simulink model "MODEL_GR2_WITH_BRAKKING"  (R2023b)
settings: Solver=VariableStepAuto  StartTime=0.0  StopTime=T_tot  RelTol=1e-3
values from neighbouring files (symbols this model uses):
  B = 0.0129    [PARAMETERS_MODEL_GR2.m]    (also in Parameters.m; Parameters_Chloe.m)
  C_dc = 15e-3    (= 0.015)    [PARAMETERS_MODEL_GR2.m]    (also in Parameters.m; Parameters_Chloe.m)
  f_grid = 50    [PARAMETERS_MODEL_GR2.m]    (also in Parameters.m; Parameters_Chloe.m)
  f_r = 50    [PARAMETERS_MODEL_GR2.m]    (also in Parameters.m; Parameters_Chloe.m)
  J = 0.2799    [PARAMETERS_MODEL_GR2.m]    (also in Parameters.m; Parameters_Chloe.m)
  Ki = Ki*Ts_w    (= 0.00645)    [PARAMETERS_MODEL_GR2.m]    (also in Parameters.m = 0.37903125; Parameters_Chloe.m = 1.04185)
  Kp = Kp + Ki*Ts_w/2    (= 210.627975)    [PARAMETERS_MODEL_GR2.m]    (also in Parameters.m = 2.463703125; Parameters_Chloe.m = 6.772025)
  L_grid = 1.5e-6    (= 1.5e-06)    [PARAMETERS_MODEL_GR2.m]    (also in Parameters.m = 2e-05; Parameters_Chloe.m = 2e-05)
  L_lr = 1.8e-3    (= 0.0018)    [PARAMETERS_MODEL_GR2.m]    (also in Parameters.m; Parameters_Chloe.m)
  L_ls = 1.8e-3    (= 0.0018)    [PARAMETERS_MODEL_GR2.m]    (also in Parameters.m; Parameters_Chloe.m)
  L_rectif = 10e-3    (= 0.01)    [PARAMETERS_MODEL_GR2.m]    (also in Parameters.m; Parameters_Chloe.m)
  N_steady = N_r    (= 1460)    [PARAMETERS_MODEL_GR2.m]    (also in Parameters.m = 1450; Parameters_Chloe.m = 1450)
  P = 4    [PARAMETERS_MODEL_GR2.m]    (also in Parameters.m; Parameters_Chloe.m)
  p = P/2    (= 2)    [PARAMETERS_MODEL_GR2.m]
  P_r = 19e3    (= 19000)    [PARAMETERS_MODEL_GR2.m]    (also in Parameters.m; Parameters_Chloe.m)
  Phi_n = V_s/w_s    [PARAMETERS_MODEL_GR2.m]    (also in Parameters.m = V_r*sqrt(2)/sqrt(3)/(2*pi*f_r); Parameters_Chloe.m = V_r*sqrt(2)/sqrt(3)/(2*pi*f_r))
  R_grid = 0.005    [PARAMETERS_MODEL_GR2.m]    (also in Parameters.m = 0.2; Parameters_Chloe.m = 0.2)
  R_r = 0.1091    [PARAMETERS_MODEL_GR2.m]    (also in Parameters.m; Parameters_Chloe.m)
  R_s = 0.0629    [PARAMETERS_MODEL_GR2.m]    (also in Parameters.m; Parameters_Chloe.m)
  Slope_down = -N_steady/(t_rampdown_end - t_rampdown_start)    (= -912.5)    [PARAMETERS_MODEL_GR2.m]
  Slope_up = N_steady/(t_rampup_end - t_rampup_start)    (= 912.5)    [PARAMETERS_MODEL_GR2.m]
  t_delay_down = 0.01*T_tot    (= 0.08)    [PARAMETERS_MODEL_GR2.m]
  t_delay_up = 0.03*T_tot    (= 0.24)    [PARAMETERS_MODEL_GR2.m]
  T_load = 0.8*T_r    (= 99.4173343149)    [PARAMETERS_MODEL_GR2.m]
  t_rampdown_end = 0.95*T_tot    (= 7.6)    [PARAMETERS_MODEL_GR2.m]
  t_rampdown_start = 0.75*T_tot    (= 6)    [PARAMETERS_MODEL_GR2.m]
  t_rampup_start = 0.05*T_tot    (= 0.4)    [PARAMETERS_MODEL_GR2.m]
  T_sat = 0.9*T_max    [PARAMETERS_MODEL_GR2.m]    (also in Parameters.m = 124.271667894; Parameters_Chloe.m = 621.358339468)
  Ts = 5e-6    (= 5e-06)    [PARAMETERS_MODEL_GR2.m]    (also in Parameters.m = 1e-05; Parameters_Chloe.m = 1e-05)
  Ts_w = 1/fs_w    (= 0.000664451827243)    [PARAMETERS_MODEL_GR2.m]    (also in Parameters.m = 0.0410256410256; Parameters_Chloe.m = 0.0149253731343)
  U_ac = 380    [PARAMETERS_MODEL_GR2.m]    (also in Parameters.m; Parameters_Chloe.m)
  V_f_in = [-f_r-1 -f_r -f_min 0 f_min f_r f_r+1]*2*pi    [PARAMETERS_MODEL_GR2.m]    (also in Parameters.m; Parameters_Chloe.m)
  V_f_out = [V_s V_s V_min V_min V_min V_s V_s]/V_s    [PARAMETERS_MODEL_GR2.m]    (also in Parameters.m = [V_r V_r V_min V_min V_min V_r V_r]/V_r; Parameters_Chloe.m = [V_r V_r V_min V_min V_min V_r V_r]/V_r)
  V_r = 400    [PARAMETERS_MODEL_GR2.m]    (also in Parameters.m; Parameters_Chloe.m)
libraries: spsDiodeLib x13, spsIGBTLib x7, spsSeriesRLCBranchLib x6, spsACVoltageSourceLib x3, spsThreePhaseVIMeasurementLib x3, spsMeanLib x2, spsRMSLib x2, simulink x2, spsAsynchronousMachineSIUnitsLib x1, spsCurrentMeasurementLib x1, spsGroundLib x1, spsThreePhaseTransformerTwoWindingsLib x1
settings Model: Creator=dimit  LastModifiedBy=User

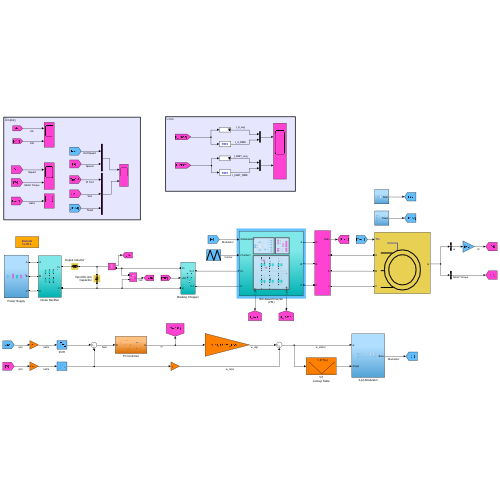
[thumbnail: Simulink's stored preview of the top-level diagram]
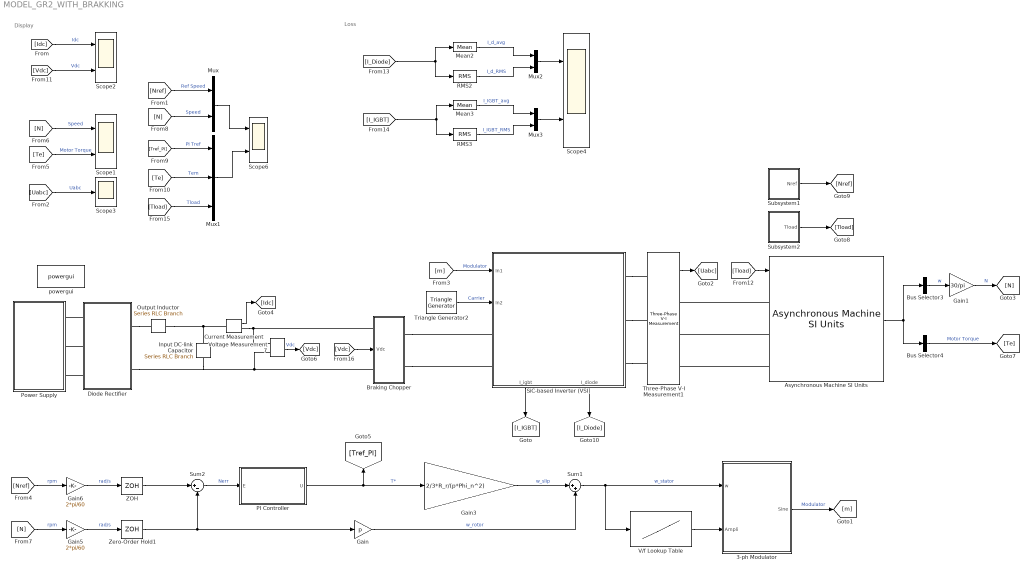
== system MODEL_GR2_WITH_BRAKKING ==
  note: Display
  note: Loss
  3-ph Modulator : Subsystem
  Asynchronous Machine SI Units : spsAsynchronousMachineSIUnitsLib/Asynchronous Machine SI Units  RotorType=Squirrel-cage  PresetModel=No  MechanicalLoad=Torque Tm  ShowDetailedParameters=on  ReferenceFrame=Rotor  Units=SI  MeasurementBus=off  NominalParameters=[P_r V_r f_r]  VoltageRatio=1  Stator=[R_s L_ls]  Rotor=[R_r L_lr]  Cage1=[0.4155 0.002066]  Cage2=[0.4168 0.0003495]  Lm=L_m  Mechanical=[J B P/2]  PolePairs=2  InitialConditions=[1 0 0 0 0 0 0 0]  SimulateSaturation=off  Saturation=[14.03593122, 27.81365428, 53.79336849, 72.68890987, 97.98006896, 148.6815601, 215.7428561, 302.9841135, 428.7778367 ; 230, 322, 414, 460, 506, 552, 598, 644, 690]  LoadFlowParameters=1492000  TsPowergui=0  TsBlock=-1  IterativeModel=Trapezoidal non iterative  IterativeDiscreteModel=Trapezoidal non iterative  Pmec=1.492e+006
  Braking Chopper : Subsystem
      settings: PortSchema="{\"entries\":[{\"content\":{\"sides\":[{\"content\":{\"connectorIds\":[\"LConn1\",\"In1\",\"LConn2\"]},\"type\":\"ConnectorPlacement.EquallySpacedRectSide\",\"uuid\":\"08066bb6-7173-482b-b457-6e49107a8511\"},{\"content\":{\"connectorIds\":[\"RConn1\",\"RConn2\"],\"side\":\"RIGHT\"},\"type\":\"ConnectorPlacement.EquallySpacedRectSide\",\"uuid\":\"28fab536-82b6-47c9-b368-73f431d395c4\"},{\"content\":{\"side\":\"TOP\"},\"type\":\"ConnectorPlacement.EquallySpacedRectSide\",\"uuid\":\"9838844e-a39c-4f91-95c1-e91ef715e2ab\"}]},\"type\":\"ConnectorPlacement.EquallySpacedConnector\",\"uuid\":\"fe40f05d-eb20-40bd-af99-b051ef6fbc42\"}],\"packageUris\":[\"http://schema.mathworks.com/mf0/Connector/R2020b\"],\"version\":\"1.0\"}"
  Bus Selector3 : BusSelector  OutputSignals=Mechanical.Rotor speed (wm)  OutputAsBus=on
  Bus Selector4 : BusSelector  OutputSignals=Mechanical.Electromagnetic torque Te (N*m)  OutputAsBus=on
  Current Measurement : spsCurrentMeasurementLib/Current Measurement  PhasorSimulation=off  OutputType=Complex  PSBequivalent=0
  Diode Rectifier : Subsystem
  Gain : Gain  Gain=p
  Gain1 : Gain  Gain=30/pi
  Gain3 : Gain  Gain=2/3*R_r/(p*Phi_n^2)
  Gain5 : Gain  Gain=2*pi/60
  Gain6 : Gain  Gain=2*pi/60
  Input DC-link Capacitor : spsSeriesRLCBranchLib/Series RLC Branch  LConnTagsString=__new0  RConnTagsString=__new0  BranchType=C  Resistance=1  Inductance=1e-3  SetiL0=off  InitialCurrent=0  Capacitance=C_dc  Setx0=off  InitialVoltage=0  Measurements=None
  Mean2 : spsMeanLib/Mean  Freq=10  Vinit=0  Ts=Ts
  Mean3 : spsMeanLib/Mean  Freq=10  Vinit=0  Ts=Ts
  Mux : Mux  Inputs=2
  Mux1 : Mux  Inputs=3
  Mux2 : Mux  Inputs=2
  Mux3 : Mux  Inputs=2
  Output Inductor : spsSeriesRLCBranchLib/Series RLC Branch  LConnTagsString=__new0  RConnTagsString=__new0  BranchType=L  Resistance=1  Inductance=L_rectif  SetiL0=off  InitialCurrent=0  Capacitance=15e-6  Setx0=off  InitialVoltage=0  Measurements=None
  PI Controller : Subsystem
  Power Supply : Subsystem
  RMS2 : spsRMSLib/RMS  TrueRMS=on  Freq=10  RMSInit=0  Ts=Ts
  RMS3 : spsRMSLib/RMS  TrueRMS=on  Freq=10  RMSInit=0  Ts=Ts
  Scope{1..2,4,6} (4 alike) : Scope  NumInputPorts=2
  Scope3 : Scope
  SiC-based Inverter (VSI) : Subsystem
      settings: PortSchema="{\"entries\":[{\"content\":{\"sides\":[{\"content\":{\"connectorIds\":[\"In1\",\"In2\",\"LConn1\",\"LConn2\"]},\"type\":\"ConnectorPlacement.EquallySpacedRectSide\",\"uuid\":\"45fc5859-179e-40d9-92a1-bdc86f2558ba\"},{\"content\":{\"connectorIds\":[\"RConn1\",\"RConn2\",\"RConn3\"],\"side\":\"RIGHT\"},\"type\":\"ConnectorPlacement.EquallySpacedRectSide\",\"uuid\":\"a0d57c1e-c527-4dbd-a036-7c0d4c1ba50f\"},{\"content\":{\"side\":\"TOP\"},\"type\":\"ConnectorPlacement.EquallySpacedRectSide\",\"uuid\":\"ae8306ed-bce6-46bd-8f47-d4ecdbdade45\"},{\"content\":{\"connectorIds\":[\"Out1\",\"Out2\"],\"side\":\"BOTTOM\"},\"type\":\"ConnectorPlacement.EquallySpacedRectSide\",\"uuid\":\"956e186d-7720-45d4-9cd3-94ca775912d4\"}]},\"type\":\"ConnectorPlacement.EquallySpacedConnector\",\"uuid\":\"758af6d4-83da-4acf-a819-436e3391a35e\"}],\"packageUris\":[\"http://schema.mathworks.com/mf0/Connector/R2020b\"],\"version\":\"1.0\"}"
  Subsystem1 : Subsystem
  Subsystem2 : Subsystem
  Sum1 : Sum  Inputs=|++
  Sum2 : Sum  Inputs=|+-
  Three-Phase V-I Measurement1 : spsThreePhaseVIMeasurementLib/Three-Phase V-I Measurement  VoltageMeasurement=phase-to-phase  SetLabelV=off  LabelV=Vabc  Vpu=off  VpuLL=off  CurrentMeasurement=no  SetLabelI=off  LabelI=Iabc  Ipu=off  Pbase=100e6  Vbase=500e3  OutputType=Complex  PhasorSimulation=off  PSBequivalent=0
  Triangle Generator2 : spsTriangleGeneratorLib/Triangle Generator  Freq=f_switch  Phase=0  Ts=0
  V/f Lookup Table : Lookup_n-D  NumberOfTableDimensions=1  BreakpointsForDimension1=V_f_in  Table=V_f_out  InternalRulePriority=Speed  RndMeth=Simplest
  Voltage Measurement7 : spsVoltageMeasurementLib/Voltage Measurement  PhasorSimulation=off  OutputType=Complex  PSBequivalent=0
  ZOH : ZeroOrderHold  SampleTime=Ts_w
  Zero-Order Hold1 : ZeroOrderHold  SampleTime=Ts_w
  powergui : spspowerguiLib/powergui  Priority=1  SimulationMode=Discrete  SampleTime=Ts  frequency=60  Iterations=50  frequencyindice=0  Pbase=100e6  ErrMax=1e-4  UnitsV=kV  UnitsW=MW  buscounter=0  FunctionMessages=off  echomessages=off  EnableUseOfTLC=off  CurrentSourceSwitches=off  DisableSnubberDevices=off  DisableRonSwitches=off  DisableVfSwitches=off  DisplayEquations=off  AutomaticDiscreteSolvers=off  SolverType=Tustin/Backward Euler (TBE)  Interpol=off  ExternalGateDelay=off  methode=off  Ts=100  x0status=blocks  SPID=on  SwTol=0  HookPort=off  NonlinearTolerance=1e-4  nMaxIteration=100  ContinueOnMaxIteration=off  RestoreLinks=warning  ResistiveCurrentMeasurement=off  Frange=[0:2:500]  Ylog=off  Xlog=on  ShowGrid=off  save=off  variable=ZData  structure=0  ZoomFFT=off  StartTime=0.0  cycles=1  DisplayStyle=1  fundamental=60  FreqAxis=off  MaxFrequency=1000  frequencyindicesteady=1  RmsSteady=1  display=off
  wires:
  [Te] -> Mux1/2  "Tem"
  Gain1/1 -> [N]  "N"
  [m] -> SiC-based Inverter (VSI)/1(In1)  "Modulator"
  [Uabc] -> Scope3/1  "Uabc"
  [Tref_PI] -> Mux1/1  "PI Tref"
  [Te] -> Scope1/2  "Motor Torque"
  Three-Phase V-I Measurement1/1 -> [Uabc]
  [Nref] -> Mux/1  "Ref Speed"
  [N] -> Mux/2  "Speed"
  Mux1/1 -> Scope6/2
  Triangle Generator2/1 -> SiC-based Inverter (VSI)/2(In2)  "Carrier"
  Mux/1 -> Scope6/1
  [N] -> Scope1/1  "Speed"
  Asynchronous Machine SI Units/1 -> Bus Selector3/1, Bus Selector4/1
  Bus Selector3/1 -> Gain1/1  "w"
  Bus Selector4/1 -> [Te]  "Motor Torque"
  Current Measurement/1 -> [Idc]
  Voltage Measurement7/1 -> [Vdc]  "Vdc"
  [Idc] -> Scope2/1  "Idc"
  [Vdc] -> Scope2/2  "Vdc"
  SiC-based Inverter (VSI)/1(I_igbt) -> [I_IGBT]
  PI Controller/1(U) -> [Tref_PI], Gain3/1  "T*"
  Sum1/1 -> V/f Lookup Table/1, 3-ph Modulator/1(w)  "w_stator"
  Zero-Order Hold1/1 -> Sum2/2, Gain/1
  ZOH/1 -> Sum2/1
  V/f Lookup Table/1 -> 3-ph Modulator/2(Ampli)
  [N] -> Gain5/1  "rpm"
  Gain6/1 -> ZOH/1  "rad/s"
  3-ph Modulator/1(Sine) -> [m]  "Modulator"
  Gain3/1 -> Sum1/1  "w_slip"
  Gain/1 -> Sum1/2  "w_rotor"
  Gain5/1 -> Zero-Order Hold1/1  "rad/s"
  [Nref] -> Gain6/1  "rpm"
  Sum2/1 -> PI Controller/1(E)  "Nerr"
  [Tload] -> Asynchronous Machine SI Units/1
  [I_IGBT] -> RMS3/1, Mean3/1
  Mean2/1 -> Mux2/1  "I_d_avg"
  Mean3/1 -> Mux3/1  "I_IGBT_avg"
  [I_Diode] -> Mean2/1, RMS2/1
  RMS2/1 -> Mux2/2  "I_d_RMS"
  SiC-based Inverter (VSI)/2(I_diode) -> [I_Diode]
  Subsystem2/1(Tload) -> [Tload]
  Subsystem1/1(Nref) -> [Nref]
  [Tload] -> Mux1/3  "Tload"
  RMS3/1 -> Mux3/2  "I_IGBT_RMS"
  Mux2/1 -> Scope4/1
  Mux3/1 -> Scope4/2
  [Vdc] -> Braking Chopper/1(Vdc)
  connections:
  SiC-based Inverter (VSI)/RConn1 -- Three-Phase V-I Measurement1/LConn1
  Asynchronous Machine SI Units/LConn3 -- Three-Phase V-I Measurement1/RConn3
  SiC-based Inverter (VSI)/RConn3 -- Three-Phase V-I Measurement1/LConn3
  Asynchronous Machine SI Units/LConn1 -- Three-Phase V-I Measurement1/RConn1
  SiC-based Inverter (VSI)/RConn2 -- Three-Phase V-I Measurement1/LConn2
  Asynchronous Machine SI Units/LConn2 -- Three-Phase V-I Measurement1/RConn2
  Input DC-link Capacitor/RConn1 -- Diode Rectifier/RConn2 -- Braking Chopper/LConn2 -- Voltage Measurement7/LConn2
  Current Measurement/RConn1 -- Voltage Measurement7/LConn1 -- Braking Chopper/LConn1
  Output Inductor/LConn1 -- Input DC-link Capacitor/LConn1 -- Current Measurement/LConn1
  Diode Rectifier/LConn1 -- Power Supply/LConn1
  Diode Rectifier/LConn2 -- Power Supply/LConn2
  Diode Rectifier/RConn1 -- Output Inductor/RConn1
  Diode Rectifier/LConn3 -- Power Supply/LConn3
  Braking Chopper/RConn1 -- SiC-based Inverter (VSI)/LConn1
  Braking Chopper/RConn2 -- SiC-based Inverter (VSI)/LConn2

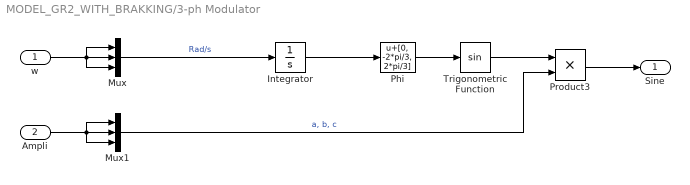
== system MODEL_GR2_WITH_BRAKKING/3-ph Modulator ==
  w : Inport
  Ampli : Inport  Port=2
  Integrator : Integrator
  Mux : Mux  Inputs=3
  Mux1 : Mux  Inputs=3
  Phi : Bias  Bias=[0, -2*pi/3, 2*pi/3]  SaturateOnIntegerOverflow=off
  Product3 : Product
  Trigonometric Function : Trigonometry
  Sine : Outport
  wires:
  Integrator/1 -> Phi/1
  Trigonometric Function/1 -> Product3/1
  Mux/1 -> Integrator/1  "Rad/s"
  Mux1/1 -> Product3/2  "a, b, c"
  Ampli/1 -> Mux1/1, Mux1/3, Mux1/2
  w/1 -> Mux/3, Mux/2, Mux/1
  Phi/1 -> Trigonometric Function/1
  Product3/1 -> Sine/1

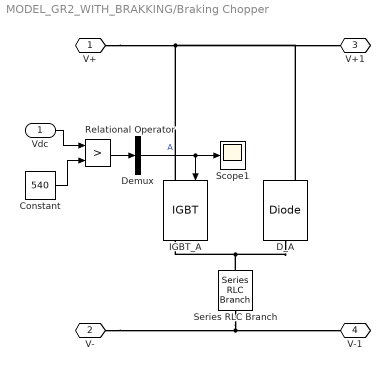
== system MODEL_GR2_WITH_BRAKKING/Braking Chopper ==
  Vdc : Inport
  Constant : Constant  Value=540
  D_A : spsDiodeLib/Diode  Ron=R_d_inv  Lon=L_on_inv  Vf=V_f_inv  IC=0  UseSnubber=0  Rs=R_snub_inv  Cs=C_snub_inv  Measurements=on
  Demux : Demux  Outputs=1
  IGBT_A : spsIGBTLib/IGBT  Ron=R_on_inv  Lon=L_on_inv  Vf=V_f_inv  Tf=1e-6  Tt=2e-6  IC=0  Rs=R_snub_inv  Cs=C_snub_inv  Measurements=on
  Relational Operator : RelationalOperator  Operator=>  OutDataTypeStr=boolean  RndMeth=Simplest  InputSameDT=off
  Scope1 : Scope
  Series RLC Branch : spsSeriesRLCBranchLib/Series RLC Branch  LConnTagsString=__new0  RConnTagsString=__new0  BranchType=R  Resistance=20  Inductance=1e-3  SetiL0=off  InitialCurrent=0  Capacitance=1e-6  Setx0=off  InitialVoltage=0  Measurements=None
  V+ : PMIOPort  Side=Left
  V- : PMIOPort  Port=2  Side=Left
  V+1 : PMIOPort  Port=3  Side=Right
  V-1 : PMIOPort  Port=4  Side=Right
  wires:
  Vdc/1 -> Relational Operator/1
  Constant/1 -> Relational Operator/2
  Relational Operator/1 -> Demux/1
  Demux/1 -> Scope1/1, IGBT_A/1  "A"
  connections:
  V+/RConn1 -- IGBT_A/LConn1 -- D_A/RConn1 -- V+1/RConn1
  V-/RConn1 -- Series RLC Branch/RConn1 -- V-1/RConn1
  Series RLC Branch/LConn1 -- D_A/LConn1 -- IGBT_A/RConn1

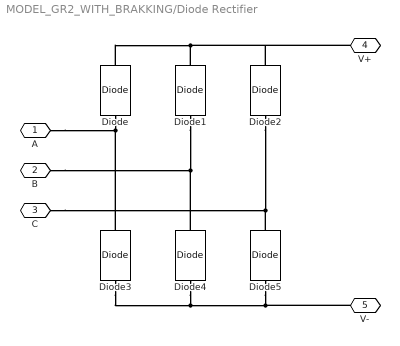
== system MODEL_GR2_WITH_BRAKKING/Diode Rectifier ==
  Diode{,1..5} (6 alike) : spsDiodeLib/Diode  Ron=R_on_rect  Lon=0  Vf=V_f_rect  IC=0  UseSnubber=0  Rs=R_snub_rect  Cs=C_snub_rect  Measurements=off
  A : PMIOPort  Side=Left
  B : PMIOPort  Port=2  Side=Left
  C : PMIOPort  Port=3  Side=Left
  V+ : PMIOPort  Port=4  Side=Right
  V- : PMIOPort  Port=5  Side=Right
  connections:
  B/RConn1 -- Diode4/RConn1 -- Diode1/LConn1
  Diode4/LConn1 -- Diode3/LConn1 -- Diode5/LConn1 -- V-/RConn1
  C/RConn1 -- Diode5/RConn1 -- Diode2/LConn1
  Diode/LConn1 -- Diode3/RConn1 -- A/RConn1
  Diode/RConn1 -- Diode1/RConn1 -- Diode2/RConn1 -- V+/RConn1

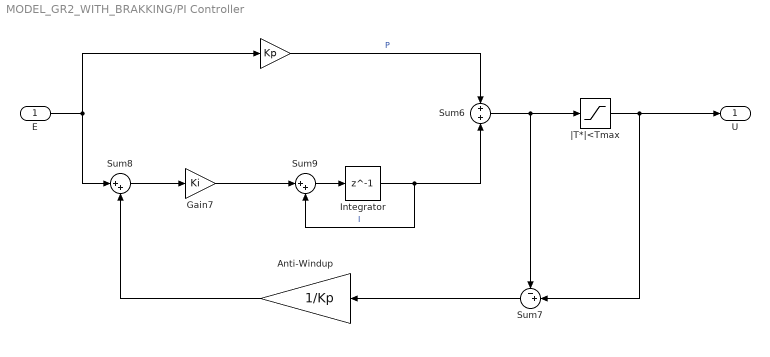
== system MODEL_GR2_WITH_BRAKKING/PI Controller ==
  E : Inport
  " " : Gain  Gain=Kp
  Anti-Windup : Gain  Gain=1/Kp
  Gain7 : Gain  Gain=Ki
  Integrator : Delay  DelayLength=1  SampleTime=Ts_w
  Sum6 : Sum
  Sum7 : Sum  Inputs=-+|
  Sum8 : Sum  Inputs=|++
  Sum9 : Sum  Inputs=|++
  |T*|<Tmax : Saturate  UpperLimit=T_sat  LowerLimit=-T_sat
  U : Outport
  wires:
  Sum8/1 -> Gain7/1
  Anti-Windup/1 -> Sum8/2
  E/1 -> Sum8/1, " "/1
  Sum6/1 -> |T*|<Tmax/1, Sum7/1
  " "/1 -> Sum6/1  "P"
  |T*|<Tmax/1 -> Sum7/2, U/1
  Integrator/1 -> Sum6/2, Sum9/2  "I"
  Sum7/1 -> Anti-Windup/1
  Gain7/1 -> Sum9/1
  Sum9/1 -> Integrator/1

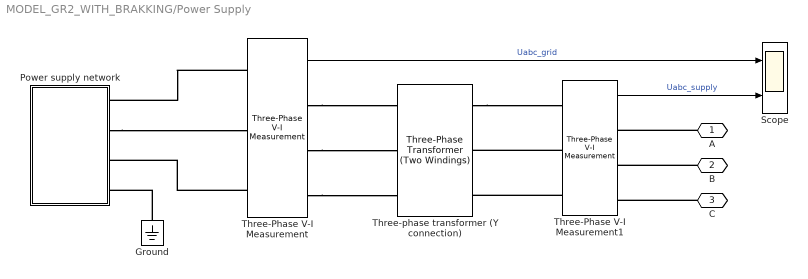
== system MODEL_GR2_WITH_BRAKKING/Power Supply ==
  Ground : spsGroundLib/Ground  LConnTagsString=a
  Power supply network : Subsystem
  Scope : Scope  NumInputPorts=2
  Three-Phase V-I Measurement : spsThreePhaseVIMeasurementLib/Three-Phase V-I Measurement  VoltageMeasurement=phase-to-phase  SetLabelV=off  LabelV=Vabc  Vpu=off  VpuLL=off  CurrentMeasurement=no  SetLabelI=off  LabelI=Iabc  Ipu=off  Pbase=100e6  Vbase=500e3  OutputType=Complex  PhasorSimulation=off  PSBequivalent=0
  Three-Phase V-I Measurement1 : spsThreePhaseVIMeasurementLib/Three-Phase V-I Measurement  VoltageMeasurement=phase-to-phase  SetLabelV=off  LabelV=Vabc  Vpu=off  VpuLL=off  CurrentMeasurement=no  SetLabelI=off  LabelI=Iabc  Ipu=off  Pbase=100e6  Vbase=500e3  OutputType=Complex  PhasorSimulation=off  PSBequivalent=0
  Three-phase transformer (Y connection) : spsThreePhaseTransformerTwoWindingsLib/Three-Phase Transformer (Two Windings)  Winding1Connection=Y  Winding2Connection=Yg  CoreType=Three single-phase transformers  SetSaturation=off  Hysteresis=off  DataFile='hysteresis'  SetInitialFlux=off  Measurements=None  UNITS=pu  NominalPower=[ 20e3 , 50 ]  Winding1=[ 380 , 0.002 , 0.08 ]  Winding2=[ 380 , 0.002 , 0.08 ]  Rm=500  Lm=500  L0=0.5  Saturation=[ 0,0 ; 0.0024,1.2 ; 1.0,1.52 ]  InitialFluxes=[ 0.8 , -0.8 , 0.7 ]  BreakLoop=off  DiscreteSolver=Trapezoidal iterative  DataType=off  TransfoNumber=1
  A : PMIOPort  Side=Left
  B : PMIOPort  Port=2  Side=Left
  C : PMIOPort  Port=3  Side=Left
  wires:
  Three-Phase V-I Measurement1/1 -> Scope/2  "Uabc_supply"
  Three-Phase V-I Measurement/1 -> Scope/1  "Uabc_grid"
  connections:
  Three-phase transformer (Y connection)/RConn1 -- Three-Phase V-I Measurement1/LConn1
  Three-Phase V-I Measurement1/LConn2 -- Three-phase transformer (Y connection)/RConn2
  Three-Phase V-I Measurement1/LConn3 -- Three-phase transformer (Y connection)/RConn3
  Three-Phase V-I Measurement/RConn1 -- Three-phase transformer (Y connection)/LConn1
  Three-Phase V-I Measurement/RConn2 -- Three-phase transformer (Y connection)/LConn2
  Three-Phase V-I Measurement/RConn3 -- Three-phase transformer (Y connection)/LConn3
  A/RConn1 -- Three-Phase V-I Measurement1/RConn1
  B/RConn1 -- Three-Phase V-I Measurement1/RConn2
  C/RConn1 -- Three-Phase V-I Measurement1/RConn3
  Three-Phase V-I Measurement/LConn1 -- Power supply network/LConn1
  Power supply network/LConn2 -- Three-Phase V-I Measurement/LConn2
  Ground/LConn1 -- Power supply network/LConn4
  Three-Phase V-I Measurement/LConn3 -- Power supply network/LConn3

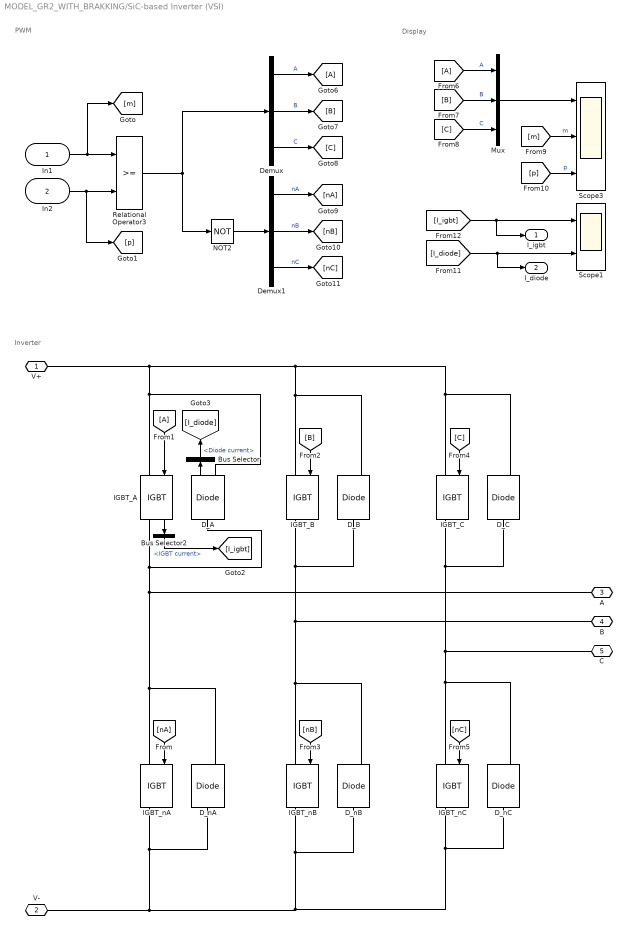
== system MODEL_GR2_WITH_BRAKKING/SiC-based Inverter (VSI) ==
  note: Display
  note: PWM
  note: Inverter
  In1 : Inport
  In2 : Inport  Port=2
  Bus Selector : BusSelector  OutputSignals=Diode current
  Bus Selector2 : BusSelector  OutputSignals=IGBT current
  D_A : spsDiodeLib/Diode  Ron=R_d_inv  Lon=L_on_inv  Vf=V_f_inv  IC=0  UseSnubber=0  Rs=R_snub_inv  Cs=C_snub_inv  Measurements=on
  D_B : spsDiodeLib/Diode  Ron=R_d_inv  Lon=L_on_inv  Vf=V_f_inv  IC=0  UseSnubber=0  Rs=R_snub_inv  Cs=C_snub_inv  Measurements=on
  D_C : spsDiodeLib/Diode  Ron=R_d_inv  Lon=L_on_inv  Vf=V_f_inv  IC=0  UseSnubber=0  Rs=R_snub_inv  Cs=C_snub_inv  Measurements=on
  D_nA : spsDiodeLib/Diode  Ron=R_d_inv  Lon=L_on_inv  Vf=V_f_inv  IC=0  UseSnubber=0  Rs=R_snub_inv  Cs=C_snub_inv  Measurements=on
  D_nB : spsDiodeLib/Diode  Ron=R_d_inv  Lon=L_on_inv  Vf=V_f_inv  IC=0  UseSnubber=0  Rs=R_snub_inv  Cs=C_snub_inv  Measurements=on
  D_nC : spsDiodeLib/Diode  Ron=R_d_inv  Lon=L_on_inv  Vf=V_f_inv  IC=0  UseSnubber=0  Rs=R_snub_inv  Cs=C_snub_inv  Measurements=on
  Demux : Demux  Outputs=3
  Demux1 : Demux  Outputs=3
  From1 : From
  From6 : From
  Goto6 : Goto
  IGBT_A : spsIGBTLib/IGBT  Ron=R_on_inv  Lon=L_on_inv  Vf=V_f_inv  Tf=1e-6  Tt=2e-6  IC=0  Rs=R_snub_inv  Cs=C_snub_inv  Measurements=on
  IGBT_B : spsIGBTLib/IGBT  Ron=R_on_inv  Lon=L_on_inv  Vf=V_f_inv  Tf=1e-6  Tt=2e-6  IC=0  Rs=R_snub_inv  Cs=C_snub_inv  Measurements=on
  IGBT_C : spsIGBTLib/IGBT  Ron=R_on_inv  Lon=L_on_inv  Vf=V_f_inv  Tf=1e-6  Tt=2e-6  IC=0  Rs=R_snub_inv  Cs=C_snub_inv  Measurements=on
  IGBT_nA : spsIGBTLib/IGBT  Ron=R_on_inv  Lon=L_on_inv  Vf=V_f_inv  Tf=1e-6  Tt=2e-6  IC=0  Rs=R_snub_inv  Cs=C_snub_inv  Measurements=on
  IGBT_nB : spsIGBTLib/IGBT  Ron=R_on_inv  Lon=L_on_inv  Vf=V_f_inv  Tf=1e-6  Tt=2e-6  IC=0  Rs=R_snub_inv  Cs=C_snub_inv  Measurements=on
  IGBT_nC : spsIGBTLib/IGBT  Ron=R_on_inv  Lon=L_on_inv  Vf=V_f_inv  Tf=1e-6  Tt=2e-6  IC=0  Rs=R_snub_inv  Cs=C_snub_inv  Measurements=on
  Mux : Mux  Inputs=3
  NOT2 : Logic  Operator=NOT  AllPortsSameDT=off  OutDataTypeStr=boolean
  Relational Operator3 : RelationalOperator  OutDataTypeStr=boolean  RndMeth=Simplest  InputSameDT=off
  Scope1 : Scope  NumInputPorts=2
  Scope3 : Scope  NumInputPorts=3
  V+ : PMIOPort  Side=Left
  V- : PMIOPort  Port=2  Side=Left
  A : PMIOPort  Port=3  Side=Right
  B : PMIOPort  Port=4  Side=Right
  C : PMIOPort  Port=5  Side=Right
  I_igbt : Outport
  I_diode : Outport  Port=2
  wires:
  [nA] -> IGBT_nA/1
  [C] -> IGBT_C/1
  [nB] -> IGBT_nB/1
  From1/1 -> IGBT_A/1
  [nC] -> IGBT_nC/1
  In2/1 -> Relational Operator3/2, [p]
  [B] -> IGBT_B/1
  In1/1 -> [m], Relational Operator3/1
  Relational Operator3/1 -> NOT2/1, Demux/1
  Demux/1 -> Goto6/1  "A"
  Demux/2 -> [B]  "B"
  Demux/3 -> [C]  "C"
  Demux1/3 -> [nC]  "nC"
  Demux1/1 -> [nA]  "nA"
  Demux1/2 -> [nB]  "nB"
  NOT2/1 -> Demux1/1
  From6/1 -> Mux/1  "A"
  [B] -> Mux/2  "B"
  [C] -> Mux/3  "C"
  Mux/1 -> Scope3/1
  [m] -> Scope3/2  "m"
  [p] -> Scope3/3  "p"
  IGBT_A/1 -> Bus Selector2/1
  D_A/1 -> Bus Selector/1
  Bus Selector/1 -> [I_diode]  "<Diode current>"
  Bus Selector2/1 -> [I_igbt]  "<IGBT current>"
  [I_diode] -> I_diode/1, Scope1/2
  [I_igbt] -> Scope1/1, I_igbt/1
  connections:
  V+/RConn1 -- D_C/RConn1 -- IGBT_C/LConn1 -- D_B/RConn1 -- IGBT_B/LConn1 -- IGBT_A/LConn1 -- D_A/RConn1
  V-/RConn1 -- D_nB/LConn1 -- IGBT_nB/RConn1 -- D_nC/LConn1 -- IGBT_nC/RConn1 -- D_nA/LConn1 -- IGBT_nA/RConn1
  A/RConn1 -- IGBT_A/RConn1 -- D_A/LConn1 -- IGBT_nA/LConn1 -- D_nA/RConn1
  IGBT_B/RConn1 -- D_B/LConn1 -- D_nB/RConn1 -- IGBT_nB/LConn1 -- B/RConn1
  IGBT_C/RConn1 -- D_C/LConn1 -- D_nC/RConn1 -- IGBT_nC/LConn1 -- C/RConn1

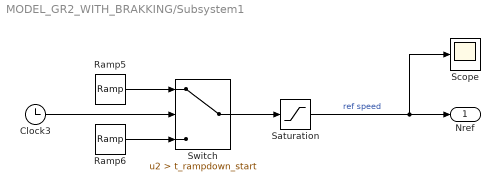
== system MODEL_GR2_WITH_BRAKKING/Subsystem1 ==
  Clock3 : Clock
  Ramp5 : simulink/Sources/Ramp  slope=Slope_down  start=t_rampdown_start  InitialOutput=N_steady
  Ramp6 : simulink/Sources/Ramp  slope=Slope_up  start=t_rampup_start  InitialOutput=0
  Saturation : Saturate  UpperLimit=N_steady  LowerLimit=0
  Scope : Scope
  Switch : Switch  Criteria=u2 > Threshold  Threshold=t_rampdown_start  SaturateOnIntegerOverflow=off  InputSameDT=off
  Nref : Outport
  wires:
  Saturation/1 -> Scope/1, Nref/1  "ref speed"
  Clock3/1 -> Switch/2
  Ramp6/1 -> Switch/3
  Switch/1 -> Saturation/1
  Ramp5/1 -> Switch/1

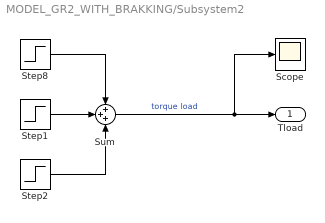
== system MODEL_GR2_WITH_BRAKKING/Subsystem2 ==
  Scope : Scope
  Step1 : Step  Time=t_rampdown_start + t_delay_down  After=-2*T_load  SampleTime=0
  Step2 : Step  Time=t_rampdown_end  After=T_load  SampleTime=0
  Step8 : Step  Time=t_rampup_start + t_delay_up  After=T_load  SampleTime=0
  Sum : Sum  Inputs=+++
  Tload : Outport
  wires:
  Sum/1 -> Scope/1, Tload/1  "torque load"
  Step8/1 -> Sum/1
  Step1/1 -> Sum/2
  Step2/1 -> Sum/3

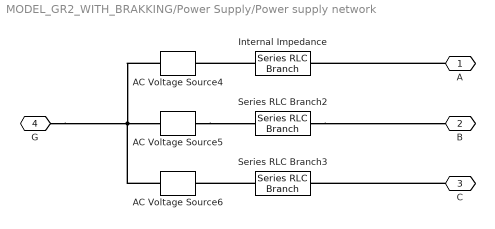
== system MODEL_GR2_WITH_BRAKKING/Power Supply/Power supply network ==
  AC Voltage Source4 : spsACVoltageSourceLib/AC Voltage Source  Amplitude=U_ac/sqrt(3)*sqrt(2)  Phase=0  Frequency=f_grid  SampleTime=0  Measurements=None  BusType=swing  Pref=10e3  Qref=0  Qmin=-inf  Qmax=+inf
  AC Voltage Source5 : spsACVoltageSourceLib/AC Voltage Source  Amplitude=U_ac/sqrt(3)*sqrt(2)  Phase=-120  Frequency=f_grid  SampleTime=0  Measurements=None  BusType=swing  Pref=10e3  Qref=0  Qmin=-inf  Qmax=+inf
  AC Voltage Source6 : spsACVoltageSourceLib/AC Voltage Source  Amplitude=U_ac/sqrt(3)*sqrt(2)  Phase=120  Frequency=f_grid  SampleTime=0  Measurements=None  BusType=swing  Pref=10e3  Qref=0  Qmin=-inf  Qmax=+inf
  Internal Impedance : spsSeriesRLCBranchLib/Series RLC Branch  LConnTagsString=__new0  RConnTagsString=__new0  BranchType=RL  Resistance=R_grid  Inductance=L_grid  SetiL0=off  InitialCurrent=0  Capacitance=15e-6  Setx0=off  InitialVoltage=0  Measurements=None
  Series RLC Branch2 : spsSeriesRLCBranchLib/Series RLC Branch  LConnTagsString=__new0  RConnTagsString=__new0  BranchType=RL  Resistance=R_grid  Inductance=L_grid  SetiL0=off  InitialCurrent=0  Capacitance=15e-6  Setx0=off  InitialVoltage=0  Measurements=None
  Series RLC Branch3 : spsSeriesRLCBranchLib/Series RLC Branch  LConnTagsString=__new0  RConnTagsString=__new0  BranchType=RL  Resistance=R_grid  Inductance=L_grid  SetiL0=off  InitialCurrent=0  Capacitance=15e-6  Setx0=off  InitialVoltage=0  Measurements=None
  A : PMIOPort  Side=Left
  B : PMIOPort  Port=2  Side=Left
  C : PMIOPort  Port=3  Side=Left
  G : PMIOPort  Port=4  Side=Left
  connections:
  A/RConn1 -- Internal Impedance/LConn1
  C/RConn1 -- Series RLC Branch3/LConn1
  AC Voltage Source5/RConn1 -- Series RLC Branch2/RConn1
  Series RLC Branch3/RConn1 -- AC Voltage Source6/RConn1
  Series RLC Branch2/LConn1 -- B/RConn1
  AC Voltage Source6/LConn1 -- G/RConn1 -- AC Voltage Source5/LConn1 -- AC Voltage Source4/LConn1
  Internal Impedance/RConn1 -- AC Voltage Source4/RConn1
